simulink library "WECSim_Lib_Body_Elements_2022b"  (R2022b)
settings: Solver=VariableStepAuto  StartTime=0.0  StopTime=10.0  RelTol=1e-3
undefined symbols (not defined in the file or in its folder): body, simu, waves, X, Y, Z
libraries: nesl_utility x24, sm_lib x21, $bdroot x12, vrlib x2
(part 1 of 4)
settings Model: Creator=kmruehl  LastModifiedBy=shusain
settings SolverCC: AlgebraicLoopSolver=TrustRegion
settings DebuggingCC: UnconnectedInputMsg=warning  UnconnectedOutputMsg=warning  UnconnectedLineMsg=warning  SFMachineParentedDataDiag=warning
settings ModelReferenceCC: EnableRefExpFcnMdlSchedulingChecks=on

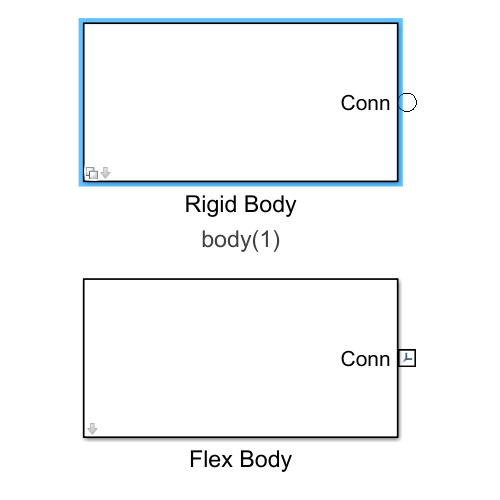
[thumbnail: Simulink's stored preview of the top-level diagram]
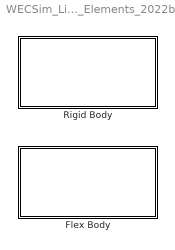
== system WECSim_Lib_Body_Elements_2022b ==
  Flex Body : Subsystem  VariantControl=(default)  mask(Flex Body){body=body(1), InputFileText=Global Reference Frame option "Use Input File" is selected., h5File=hydroData/*.h5, geometryFile=geometry/*.stl, mass=0, inertia=0 0 0, nonHydro=0, nonlinearHydro=0, centerGravity=0 0 0, centerBuoyancy=0 0 0, dof=, volume=0, flex=1, displacement=0 0 0, axis=0 1 0, angle=0, option=0, cd=0 0 0, ca=0 0 0, area=0 0 0, VME=0, rgME=0 0 0, z=0 0 1}
      mask prompts: body "Body Number:"; mass "Body Mass [kg]:"; inertia "MoI [kg*m^2]:"; nonHydro "Nonhydro Body"; nonlinearHydro "Nonlinear Hydrodynamics"; centerGravity "Center of gravity [m]"; centerBuoyancy "Center of buoyancy [m]"; dof "Degrees of freedom"; volume "Displaced Volume [m^3]"; flex "Flexible Body"; displacement "Initial Linear Displacement"; axis "Initial Angular Displacement Axis"; angle "Initial Angular Displacement"; option "On/Off"; cd "Drag coefficient"; ca "Added mass coefficient"; area "Characteristic Area"; VME "Characteristic Volume"; rgME "Point of Application"; z "Z axis"
      mask help:
      | A Flex Body may contain generalized body modes that account for various bending, shear or other deformation modes. The BEM output must contain data for these additional DOFs.
      |
      | The variable name input below must be 'body(i)' where i=1,2,...
      | body(i) must be defined in the input file with the following fields:
      |
      |     .flexHydroBody = 1 (required)
      |             Float.
      |             Flag that creates a flex body. Set equal to 1 if the BEM data contains more than 6 degrees of freedom.
      |     .filename (required)
      |             String.
      |             The file path specifying the .h5 file for the body.
      |     .mass (required)
      |             Float or string.
      |             The translational interia or mass of the body in kg. If a string, the value must be 'equilibrium'. Default = [ ]
      |     .momOfIntertia (required)
      |             3x1 vector [Ixx Iyy Izz].
      |             Rotational intertia of the body in kg*m^2. Default = [ ]
      |     .geometryFile (optional)
      |             String
      |             Path to the geometry file of the body (.stl). Required for nonlinear hydrodynamics or visualization. Default = [ ]
      mask init:
      | if exist('body','var')
      |     % geometry file name
      |     h=[gcb '/Structure/Body Properties'];
      |     geomFile=body.geometryFile;
      |     set_param(h,'ExtGeomFileName',geomFile);
      |     geomType='STL';
      |     % split version e.g. '9.10.0.16028 (R2021a)' into 9, 10, 0, NaN.
      |     % cannot compare str2double('9.10') because it becomes '9.1' 
      |     ver=split(version,'.');
      |     ver=str2double(ver(1:3));
      |     if ver(1) < 9 || (ver(1) == 9 && ver(2) < 6)
      |        set_param(h,'ExtGeomFileType',geomType);
      |     end
      |     % toWorkSpace: outputs
      |     h=[gcb '/To Workspace'];
      |     responseName=['body' num2str(body.number) '_out'];
      |     set_param(h,'VariableName',responseName);
      |     % toWorkSpace: hydrostatic pressures
      |     h=[gcb '/Hydrostatic Restoring Force Calculation/Hydrostatic Restoring Force Calculation/Linear and Nonlinear Restoring Force Variant Subsystem/Nonlinear Hydrostatic Restoring Force/To Workspace1'];
      |     responseName=['body' num2str(body.number) '_hspressure_out'];
      |     set_param(h,'VariableName',responseName); 
      |     % toWorkSpace: wave pressures (nonlinear Froude-Krylov)
      |     h=[gcb '/Wave Diffraction and Excitation Force Calculation/Wave Diffraction and Excitation Force Calculation/Nonlinear FK Force Variant Subsystem/With Nonlinear FroudeKrylov Force/To Workspace'];
      |     responseName=['body' num2str(body.number) '_wavenonlinearpressure_out'];
      |     set_param(h,'VariableName',responseName);
      |     % toWorkSpace: wave pressures (linear Froude-Krylov)
      |     h=[gcb '/Wave Diffraction and Excitation Force Calculation/Wave Diffraction and Excitation Force Calculation/Nonlinear FK Force Variant Subsystem/With Nonlinear FroudeKrylov Force/To Workspace1'];
      |     responseName=['body' num2str(body.number) '_wavelinearpressure_out'];
      |     set_param(h,'VariableName',responseName);
      |     % position: GoTo 
      |     h=[gcb '/Goto'];
      |     responseName=['disp' num2str(body.number)];
      |     set_param(h,'GotoTag',responseName);
      |     % position: From
      |     h=[gcb '/From'];
      |     responseName=['disp' num2str(body.number)];
      |     set_param(h,'GotoTag',responseName);
      |     % velocity: GoTo 
      |     h=[gcb '/Goto1'];
      |     responseName=['vel' num2str(body.number)];
      |     set_param(h,'GotoTag',responseName);
      |     % velocity: From 
      |     h=[gcb '/From1'];
      |     responseName=['vel' num2str(body.number)];
      |     set_param(h,'GotoTag',responseName);
      |     % acceleration: GoTo 
      |     h=[gcb '/Goto2'];
      |     responseName=['acc' num2str(body.number)];
      |     set_param(h,'GotoTag',responseName);
      |     % acceleration: From 
      |     h=[gcb '/From2'];
      |     responseName=['acc' num2str(body.number)];
      |     set_param(h,'GotoTag',responseName);
      |     %%
      |     % Flex Body Morison Element: Off
      |     h = [gcb '/Morrison Element and Viscous Damping Force Calculation/Morison Element and Viscous Damping Force Calculation/Morison Element Variant Subsystem/Morison Element Off'];
      |     responseName = ['sv_b' num2str(body.number) '_MEOff'];
      |     set_param(h,'VariantControl',responseName);
      |     %%
      |     % Flex Body Morison Element: On
      |     h = [gcb '/Morrison Element and Viscous Damping Force Calculation/Morison Element and Viscous Damping Force Calculation/Morison Element Variant Subsystem/Morison Element On'];
      |     responseName = ['sv_b' num2str(body.number) '_MEOn'];
      |     set_param(h,'VariantControl',responseName);
      |     %%
      |     % Flex Body Nonlinear FroudeKrylov Force: Off
      |     h = [gcb '/Wave Diffraction and Excitation Force Calculation/Wave Diffraction and Excitation Force Calculation/Nonlinear FK Force Variant Subsystem/No Nonlinear FroudeKrylov Force'];
      |     responseName = ['sv_b' num2str(body.number) '_linearHydro'];
      |     set_param(h,'VariantControl',responseName);
      |     %%
      |     % Flex Body Nonlinear FroudeKrylov Force: On
      |     h = [gcb '/Wave Diffraction and Excitation Force Calculation/Wave Diffraction and Excitation Force Calculation/Nonlinear FK Force Variant Subsystem/With Nonlinear FroudeKrylov Force'];
      |     responseName = ['sv_b' num2str(body.number) '_nonlinearHydro'];
      |     set_param(h,'VariantControl',responseName);
      |     %%
      |     % Flex Body Nonlinear Restoring: Off
      |     h = [gcb '/Hydrostatic Restoring Force Calculation/Hydrostatic Restoring Force Calculation/Linear and Nonlinear Restoring Force Variant Subsystem/Linear Hydrostatic Restoring Force'];
      |     responseName = ['sv_b' num2str(body.number) '_linearHydro'];
      |     set_param(h,'VariantControl',responseName);
      |     %%
      |     % Flex Body Nonlinear Restoring: On
      |     h = [gcb '/Hydrostatic Restoring Force Calculation/Hydrostatic Restoring Force Calculation/Linear and Nonlinear Restoring Force Variant Subsystem/Nonlinear Hydrostatic Restoring Force'];
      |     responseName = ['sv_b' num2str(body.number) '_nonlinearHydro'];
      |     set_param(h,'VariantControl',responseName);
      |     %%
      |     % Flex Body Nonlinear FroudeKrylov or Restoring: Instantaneous Free Surface
      |     h = [gcb '/Nonlinear Wave Elevation/Linear or Instantaneous Free Surface/Instantaneous Water Free Surface'];
      |     responseName = ['sv_b' num2str(body.number) '_instFS'];
      |     set_param(h,'VariantControl',responseName);
      |     %%
      |     % Flex Body Nonlinear FroudeKrylov or Restoring: Mean Free Surface
      |     h = [gcb '/Nonlinear Wave Elevation/Linear or Instantaneous Free Surface/Mean Water Free Surface'];
      |     responseName = ['sv_b' num2str(body.number) '_meanFS'];
      |     set_param(h,'VariantControl',responseName);
      |     %%
      | end
      mask Help:
      | A Flex Body may contain generalized body modes that account for various bending, shear or other deformation modes. The BEM output must contain data for these additional DOFs.
      | 
      | The variable name input below must be 'body(i)' where i=1,2,...
      | body(i) must be defined in the input file with the following fields:
      | 
      |     .flexHydroBody = 1 (required)
      |             Float.
      |             Flag that creates a flex body. Set equal to 1 if the BEM data contains more than 6 degrees of freedom.
      |     .filename (required)
      |             String.
      |             The file path specifying the .h5 file for the body.
      |     .mass (required)
      |             Float or string.
      |             The translational interia or mass of the body in kg. If a string, the value must be 'equilibrium'. Default = [ ]
      |     .momOfIntertia (required)
      |             3x1 vector [Ixx Iyy Izz].
      |             Rotational intertia of the body in kg*m^2. Default = [ ]
      |     .geometryFile (optional)
      |             String
      |             Path to the geometry file of the body (.stl). Required for nonlinear hydrodynamics or visualization. Default = [ ]
      mask TypeOptions nonHydro: 0 | 1 | 2
      mask Callback nonHydro: bodyClassCallback(gcbh)
      mask TypeOptions nonlinearHydro: 0 | 1 | 2
      mask TypeOptions flex: 0 | 1
      mask TypeOptions option: 0 | 1 | 2
      mask Callback option: bodyClassCallback(gcbh)
      mask DialogControl CustomParameterGroup Prompt: Custom Parameters
      mask DialogControl std_opts Prompt: Standard Options
      mask DialogControl H5button Prompt: Select .h5 File
      mask DialogControl H5button Callback: h5ButtonCallback(gcbh)
      mask DialogControl STLbutton Prompt: Select .stl File
      mask DialogControl STLbutton Callback: stlButtonCallback(gcbh)
      mask DialogControl inertia Tooltip: Moment of Inertia
      mask DialogControl initial Prompt: Initial Displacement
      mask DialogControl morisonElement Prompt: Morison Element
      mask DialogControl rgME Tooltip: The vector from the body COG to point of application for the Morison Element
      mask DialogControl z Tooltip: The unit normal vector center axis of the Morison Element
  Rigid Body : Subsystem  Variant=on  AllowZeroVariantControls=on  mask(Rigid Body){body=body(1), InputFileText=Global Reference Frame option "Use Input File" is selected., h5File=hydroData/*.h5, geometryFile=geometry/*.stl, mass=0, inertia=0 0 0, nonHydro=0, nonlinearHydro=0, centerGravity=0 0 0, centerBuoyancy=0 0 0, dof=6, volume=0, flex=0, displacement=0 0 0, axis=0 1 0, angle=0, option=0, cd=0 0 0, ca=0 0 0, area=0 0 0, VME=0, rgME=0 0 0, z=0 0 1}
      mask prompts: body "Body Number:"; mass "Body Mass [kg]:"; inertia "MoI [kg*m^2]:"; nonHydro "Nonhydro Body"; nonlinearHydro "Nonlinear Hydrodynamics"; centerGravity "Center of gravity [m]"; centerBuoyancy "Center of buoyancy [m]"; dof "Degrees of freedom"; volume "Displaced Volume [m^3]"; flex "Flexible Body"; displacement "Initial Linear Displacement"; axis "Initial Angular Displacement Axis"; angle "Initial Angular Displacement"; option "On/Off"; cd "Drag coefficient"; ca "Added mass coefficient"; area "Characteristic Area"; VME "Characteristic Volume"; rgME "Point of Application"; z "Z axis"
      mask help:
      | A rigid body has no generalized body modes. It can be a standard hydrodynamic body, a drag body, or a non-hydrodynamic body.
      |
      | The variable name input below must be 'body(i)' where i=1,2,...
      | body(i) must be defined in the input file with the fields appropriate to each variant.
      mask init:
      | if exist('body','var')
      |     %%
      |     % Hydro Body
      |     h = [gcb '/Hydrodynamic Body'];
      |     responseName = ['sv_b' num2str(body.number) '_hydroBody'];
      |     set_param(h,'VariantControl',responseName);
      |     %%
      |     % Hydro Body Morison Element: Off
      |     h = [gcb '/Hydrodynamic Body/Morison Element and Viscous Damping Force Calculation/Morison Element Variant Subsystem/Morison Element Off'];
      |     responseName = ['sv_b' num2str(body.number) '_MEOff'];
      |     set_param(h,'VariantControl',responseName);
      |     %%
      |     % Hydro Body Morison Element: On
      |     h = [gcb '/Hydrodynamic Body/Morison Element and Viscous Damping Force Calculation/Morison Element Variant Subsystem/Morison Element On'];
      |     responseName = ['sv_b' num2str(body.number) '_MEOn'];
      |     set_param(h,'VariantControl',responseName);
      |     %%
      |     % Hydro Body Nonlinear Froude Krylov Force: Off
      |     h = [gcb '/Hydrodynamic Body/Wave Diffraction and Excitation Force Calculation/Nonlinear FK Force Variant Subsystem/No Nonlinear FroudeKrylov Force'];
      |     responseName = ['sv_b' num2str(body.number) '_linearHydro'];
      |     set_param(h,'VariantControl',responseName);
      |     %%
      |     % Hydro Body Nonlinear Froude Krylov Force: On
      |     h = [gcb '/Hydrodynamic Body/Wave Diffraction and Excitation Force Calculation/Nonlinear FK Force Variant Subsystem/With Nonlinear FroudeKrylov Force'];
      |     responseName = ['sv_b' num2str(body.number) '_nonlinearHydro'];
      |     set_param(h,'VariantControl',responseName);
      |     %%
      |     % Hydro Body Nonlinear Restoring: Off
      |     h = [gcb '/Hydrodynamic Body/Hydrostatic Restoring Force Calculation/Linear and Nonlinear Restoring Force Variant Subsystem/Linear Hydrostatic Restoring Force'];
      |     responseName = ['sv_b' num2str(body.number) '_linearHydro'];
      |     set_param(h,'VariantControl',responseName);
      |     %%
      |     % Hydro Body Nonlinear Restoring: On
      |     h = [gcb '/Hydrodynamic Body/Hydrostatic Restoring Force Calculation/Linear and Nonlinear Restoring Force Variant Subsystem/Nonlinear Hydrostatic Restoring Force'];
      |     responseName = ['sv_b' num2str(body.number) '_nonlinearHydro'];
      |     set_param(h,'VariantControl',responseName);
      |     %%
      |     
      |     % Hydro Body Regular Excitation Passive Yaw: Off
      |     h = [gcb '/Hydrodynamic Body/Wave Diffraction and Excitation Force Calculation/Linear Wave Excitation Force Variant Subsystem'];
      |     responseName = ['regularWaves_b' num2str(body.number)];
      |     set_param(h,'VariantControl',responseName);
      |     %%
      |     % Hydro Body Regular Excitation Passive Yaw: On
      |     h = [gcb '/Hydrodynamic Body/Wave Diffraction and Excitation Force Calculation/Linear Wave Excitation Force Variant Subsystem'];
      |     responseName = ['sv_regularWavesNonLinYaw_b' num2str(body.number)];
      |     set_param(h,'VariantControl',responseName);
      |     %%    
      |     % Hydro Body Irregular Excitation Passive Yaw: Off
      |     h = [gcb '/Hydrodynamic Body/Wave Diffraction and Excitation Force Calculation/Linear Wave Excitation Force Variant Subsystem'];
      |     responseName = ['sv_irregularWaves_b' num2str(body.number)];
      |     set_param(h,'VariantControl',responseName);
      |     %%
      |     % Hydro Body Irregular Excitation Passive Yaw: On
      |     h = [gcb '/Hydrodynamic Body/Wave Diffraction and Excitation Force Calculation/Linear Wave Excitation Force Variant Subsystem'];
      |     responseName = ['sv_irregularWavesNonLinYaw_b' num2str(body.number)];
      |     set_param(h,'VariantControl',responseName);
      |     %%        
      |     
      |     % Hydro Body Nonlinear Froude Krylov or Restoring: Instantaneous Free Surface
      |     h = [gcb '/Hydrodynamic Body/Nonlinear Wave Elevation/Linear or Instantaneous Free Surface/Instantaneous Water Free Surface'];
      |     responseName = ['sv_b' num2str(body.number) '_instFS'];
      |     set_param(h,'VariantControl',responseName);
      |     %%
      |     % Hydro Body Nonlinear Froude Krylov or Restoring: Mean Free Surface
      |     h = [gcb '/Hydrodynamic Body/Nonlinear Wave Elevation/Linear or Instantaneous Free Surface/Mean Water Free Surface'];
      |     responseName = ['sv_b' num2str(body.number) '_meanFS'];
      |     set_param(h,'VariantControl',responseName);
      |     %%
      |     % Non-Hydro Body
      |     h = [gcb '/Non-Hydro Body'];
      |     responseName = ['sv_b' num2str(body.number) '_nonHydroBody'];
      |     set_param(h,'VariantControl',responseName);
      |     %%
      |     % Drag Body
      |     h = [gcb '/Drag Body'];
      |     responseName = ['sv_b' num2str(body.number) '_dragBody'];
      |     set_param(h,'VariantControl',responseName);
      |     %%
      |     % Drag Body Morison Element: Off
      |     h = [gcb '/Drag Body/Morison Element and Viscous Damping Force Calculation/Morison Element Variant Subsystem/Morison Element Off'];
      |     responseName = ['sv_b' num2str(body.number) '_MEOff'];
      |     set_param(h,'VariantControl',responseName);
      |     %%
      |     % Drag Body Morison Element: On
      |     h = [gcb '/Drag Body/Morison Element and Viscous Damping Force Calculation/Morison Element Variant Subsystem/Morison Element On'];
      |     responseName = ['sv_b' num2str(body.number) '_MEOn'];
      |     set_param(h,'VariantControl',responseName);
      |     %%
      |     % Set zero active variant controls to prevent label issue
      |     set_param(gcb,'AllowZeroVariantControls','on');
      | end
      | clear bc h geomFile responseName
      settings: AttributesFormatString=%<body>
      mask Help:
      | A rigid body has no generalized body modes. It can be a standard hydrodynamic body, a drag body, or a non-hydrodynamic body.
      | 
      | The variable name input below must be 'body(i)' where i=1,2,...
      | body(i) must be defined in the input file with the fields appropriate to each variant.
      mask TypeOptions nonHydro: 0 | 1 | 2
      mask Callback nonHydro: bodyClassCallback(gcbh)
      mask TypeOptions nonlinearHydro: 0 | 1 | 2
      mask TypeOptions flex: 0 | 1
      mask TypeOptions option: 0 | 1 | 2
      mask Callback option: bodyClassCallback(gcbh)
      mask DialogControl CustomParameterGroup Prompt: Custom Parameters
      mask DialogControl std_opts Prompt: Standard Options
      mask DialogControl H5button Prompt: Select .h5 File
      mask DialogControl H5button Callback: h5ButtonCallback(gcbh)
      mask DialogControl STLbutton Prompt: Select .stl File
      mask DialogControl STLbutton Callback: stlButtonCallback(gcbh)
      mask DialogControl inertia Tooltip: Moment of Inertia
      mask DialogControl initial Prompt: Initial Displacement
      mask DialogControl morisonElement Prompt: Morison Element
      mask DialogControl rgME Tooltip: The vector from the body COG to point of application for the Morison Element
      mask DialogControl z Tooltip: The unit normal vector center axis of the Morison Element

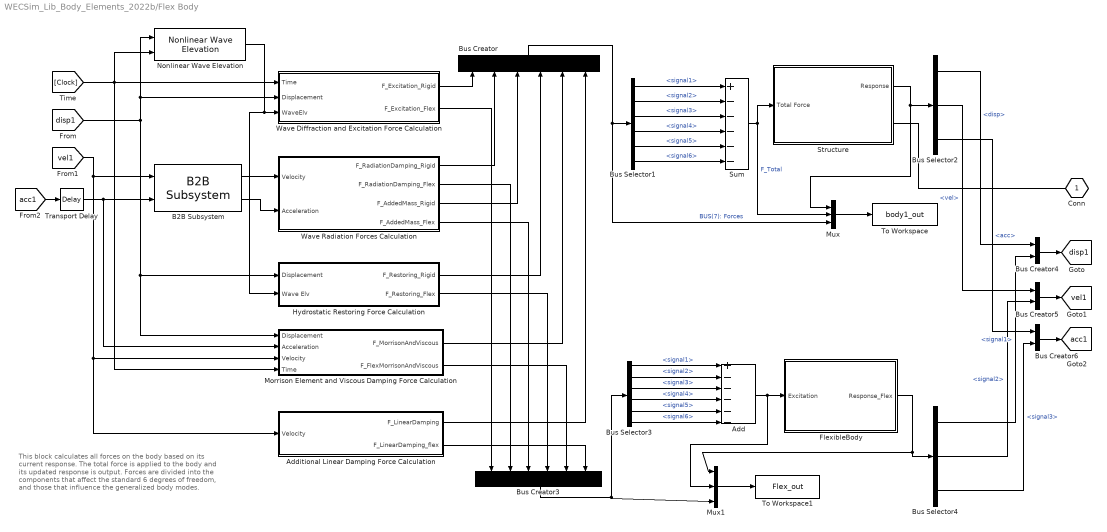
== system WECSim_Lib_Body_Elements_2022b/Flex Body ==
  note: This block calculates all forces on the body based on its current response. The total force is applied to the body and its updated response is output.
      |
      | Forces are divided into the components that affect the standard 6 degrees of freedom, and those that influence the generalized body modes.
  Add : Sum  Inputs=+-----
  Additional Linear Damping Force Calculation : Subsystem
  B2B Subsystem : $bdroot/Rigid Body/Hydrodynamic Body/B2B Subsystem  SystemSampleTime=-1  Latency=0  AutoFrameSizeCalculation=off
  Bus Creator : BusCreator  Inputs=6
  Bus Creator3 : BusCreator  Inputs=6
  Bus Creator4 : BusCreator  Inputs=2
  Bus Creator5 : BusCreator  Inputs=2
  Bus Creator6 : BusCreator  Inputs=2
  Bus Selector1 : BusSelector  OutputSignals=signal1,signal2,signal3,signal4,signal5,signal6
  Bus Selector2 : BusSelector  OutputSignals=disp,vel,acc
  Bus Selector3 : BusSelector  OutputSignals=signal1,signal2,signal3,signal4,signal5,signal6
  Bus Selector4 : BusSelector  OutputSignals=signal1,signal2,signal3
  FlexibleBody : Subsystem
  Hydrostatic Restoring Force Calculation : Subsystem
  Morrison Element and Viscous Damping Force Calculation : Subsystem
  Mux : Mux  Inputs=3
  Mux1 : Mux  Inputs=3
  Nonlinear Wave Elevation : $bdroot/Rigid Body/Hydrodynamic Body/Nonlinear Wave Elevation  SystemSampleTime=simu.nonlinearDt  Latency=0  AutoFrameSizeCalculation=off
  Structure : Subsystem
  Sum : Sum  Inputs=+-----
  To Workspace : ToWorkspace  VariableName=body1_out  SaveFormat=Structure With Time  SampleTime=simu.dtOut
  To Workspace1 : ToWorkspace  VariableName=Flex_out  SaveFormat=Structure With Time  SampleTime=simu.dtOut
  Transport Delay : TransportDelay  DelayTime=10e-8
  Wave Diffraction and Excitation Force Calculation : Subsystem
  Wave Radiation Forces Calculation : Subsystem
  Conn : PMIOPort  Side=Right
  tag scope: acc1=global, disp1=global, vel1=global
  wires:
  Bus Creator/1 -> Mux/3, Bus Selector1/1  "BUS(7): Forces"
  Structure/1(Response) -> Mux/1, Bus Selector2/1
  Sum/1 -> Mux/2, Structure/1(Total Force)  "F_Total"
  Mux/1 -> To Workspace/1
  Bus Selector1/4 -> Sum/4  "<signal4>"
  Bus Selector1/3 -> Sum/3  "<signal3>"
  Bus Selector1/5 -> Sum/5  "<signal5>"
  Bus Selector1/2 -> Sum/2  "<signal2>"
  Bus Selector1/1 -> Sum/1  "<signal1>"
  Bus Selector1/6 -> Sum/6  "<signal6>"
  [vel1] -> Additional Linear Damping Force Calculation/1(Velocity), Morrison Element and Viscous Damping Force Calculation/3(Velocity), B2B Subsystem/1
  B2B Subsystem/2 -> Wave Radiation Forces Calculation/2(Acceleration)
  B2B Subsystem/1 -> Wave Radiation Forces Calculation/1(Velocity)
  [disp1] -> Nonlinear Wave Elevation/1, Wave Diffraction and Excitation Force Calculation/2(Displacement), Morrison Element and Viscous Damping Force Calculation/1(Displacement), Hydrostatic Restoring Force Calculation/1(Displacement)
  Nonlinear Wave Elevation/1 -> Hydrostatic Restoring Force Calculation/2(Wave Elv), Wave Diffraction and Excitation Force Calculation/3(WaveElv)
  Hydrostatic Restoring Force Calculation/1(F_Restoring_Rigid) -> Bus Creator/4
  Wave Radiation Forces Calculation/1(F_RadiationDamping_Rigid) -> Bus Creator/2
  Wave Diffraction and Excitation Force Calculation/1(F_Excitation_Rigid) -> Bus Creator/1
  Wave Radiation Forces Calculation/3(F_AddedMass_Rigid) -> Bus Creator/3
  [Clock] -> Nonlinear Wave Elevation/2, Morrison Element and Viscous Damping Force Calculation/4(Time), Wave Diffraction and Excitation Force Calculation/1(Time)
  Mux1/1 -> To Workspace1/1
  Wave Diffraction and Excitation Force Calculation/2(F_Excitation_Flex) -> Bus Creator3/1
  Wave Radiation Forces Calculation/2(F_RadiationDamping_Flex) -> Bus Creator3/2
  Wave Radiation Forces Calculation/4(F_AddedMass_Flex) -> Bus Creator3/3
  Bus Creator3/1 -> Bus Selector3/1, Mux1/3
  Bus Selector3/1 -> Add/1  "<signal1>"
  Bus Selector3/2 -> Add/2  "<signal2>"
  Bus Selector3/3 -> Add/3  "<signal3>"
  Bus Selector3/4 -> Add/4  "<signal4>"
  Add/1 -> Mux1/2, FlexibleBody/1(Excitation)
  FlexibleBody/1(Response_Flex) -> Bus Selector4/1, Mux1/1
  Bus Selector4/1 -> Bus Creator4/2  "<signal1>"
  Bus Selector4/2 -> Bus Creator5/2  "<signal2>"
  Bus Selector4/3 -> Bus Creator6/2  "<signal3>"
  Additional Linear Damping Force Calculation/1(F_LinearDamping) -> Bus Creator/6
  Morrison Element and Viscous Damping Force Calculation/2("F_FlexMorrisonAndViscous ") -> Bus Creator3/5
  Bus Selector3/5 -> Add/5  "<signal5>"
  Additional Linear Damping Force Calculation/2(F_LinearDamping_flex) -> Bus Creator3/6
  Bus Selector3/6 -> Add/6  "<signal6>"
  Bus Selector2/1 -> Bus Creator4/1  "<disp>"
  Bus Creator4/1 -> [disp1]
  Bus Creator5/1 -> [vel1]
  Bus Creator6/1 -> [acc1]
  Bus Selector2/2 -> Bus Creator5/1  "<vel>"
  Bus Selector2/3 -> Bus Creator6/1  "<acc>"
  Hydrostatic Restoring Force Calculation/2(F_Restoring_Flex) -> Bus Creator3/4
  Morrison Element and Viscous Damping Force Calculation/1(F_MorrisonAndViscous) -> Bus Creator/5
  [acc1] -> Transport Delay/1
  Transport Delay/1 -> B2B Subsystem/2, Morrison Element and Viscous Damping Force Calculation/2(Acceleration)
  connections:
  Conn/RConn1 -- Structure/RConn1

== system WECSim_Lib_Body_Elements_2022b/Rigid Body ==
  note: 1) Add Subsystem or Model blocks as valid variant choices.
      | 2) You cannot connect blocks at this level. At simulation, connectivity is automatically
      | determined, based on the active variant and port name matching.
  Drag Body : Subsystem  VariantControl=sv_b1_dragBody  mask(Drag Body){body=body}
      mask prompts: body "Body Name:"
      mask help:
      | A drag body contains six degrees of freedom in x, y, z and Mx, My, Mz. It contains a buoyant force, linear damping force, and Morison Element and viscous forces. It is not influenced by wave excitation, radiation damping or radiation added mass.
      |
      | The variable name input below must be 'body(i)' where i=1,2,...
      | body(i) must be defined in the input file with the following fields:
      |
      |     .mass (required)
      |             Float or string.
      |             The translational interia or mass of the body in kg. If a string, the value must be 'equilibrium'. Default = [ ]
      |     .momOfIntertia (required)
      |             3x1 vector [Ixx Iyy Izz].
      |             Rotational intertia of the body in kg*m^2. Default = [ ]
      |     .filename (required)
      |             String.
      |             The file path specifying the .h5 file for the body.
      |     .name (optional)
      |             String.
      |             Specifies the body name. Default = [ ]
      |     .cg (optional)
      |             3x1 float vector [x y z]
      |     .cb (optional)
      |             3x1 float vector [x y z]
      |             Body center of buoyancy in m. Default = [ ].
      |     .dispVol (optional)
      |             Float.
      |             Displaced volume at the equilibrium position in m^3. Default = [ ]
      |     .geometryFile (optional)
      |             String
      |             Path to the geometry file of the body (.stl). Required for nonlinear hydrodynamics or visualization. Default = [ ]
      mask init:
      | if exist('body','var')
      |     % geometry file name
      |     h=[gcb '/Structure/Body Properties'];
      |     geomFile=body.geometryFile;
      |     set_param(h,'ExtGeomFileName',geomFile);
      |     geomType='STL';
      |     % split version e.g. '9.10.0.16028 (R2021a)' into 9, 10, 0, NaN.
      |     % cannot compare str2double('9.10') because it becomes '9.1' 
      |     ver=split(version,'.');
      |     ver=str2double(ver(1:3));
      |     if ver(1) < 9 || (ver(1) == 9 && ver(2) < 6)
      |        set_param(h,'ExtGeomFileType',geomType);
      |     end
      |     % toWorkSpace: outputs
      |     h=[gcb '/To Workspace'];
      |     responseName=['body' num2str(body.number) '_out'];
      |     set_param(h,'VariableName',responseName);
      |     % position GoTo 
      |     h=[gcb '/Goto'];
      |     responseName=['disp' num2str(body.number)];
      |     set_param(h,'GotoTag',responseName);
      |     % position From
      |     h=[gcb '/From'];
      |     responseName=['disp' num2str(body.number)];
      |     set_param(h,'GotoTag',responseName);
      |     % velocity GoTo 
      |     h=[gcb '/Goto1'];
      |     responseName=['vel' num2str(body.number)];
      |     set_param(h,'GotoTag',responseName);
      |     % velocity From 
      |     h=[gcb '/From1'];
      |     responseName=['vel' num2str(body.number)];
      |     set_param(h,'GotoTag',responseName);
      |     % acceleration GoTo 
      |     h=[gcb '/Goto2'];
      |     responseName=['acc' num2str(body.number)];
      |     set_param(h,'GotoTag',responseName);
      |     % acceleration From 
      |     h=[gcb '/From2'];
      |     responseName=['acc' num2str(body.number)];
      |     set_param(h,'GotoTag',responseName);
      | end
  Hydrodynamic Body : Subsystem  VariantControl=sv_b1_hydroBody  mask(Hydrodynamic Body){body=body, waveGroup=waves.waveGroup}
      mask prompts: body "Body Name:"; waveGroup "Wave Group:"
      mask help:
      | A Hydrodynamic Body contains six degrees of freedom in x, y, z and Mx, My, Mz. All wave forces interact with a hydrodynamic body.
      |
      | The variable name input below must be 'body(i)' where i=1,2,...
      | body(i) must be defined in the input file with the following fields:
      |
      |     .filename (required)
      |             String.
      |             The file path specifying the .h5 file for the body.
      |     .mass (required)
      |             Float or string.
      |             The translational interia or mass of the body in kg. If a string, the value must be 'equilibrium'. Default = [ ]
      |     .momOfIntertia (required)
      |             3x1 vector [Ixx Iyy Izz].
      |             Rotational intertia of the body in kg*m^2. Default = [ ]
      |     .geometryFile (optional)
      |             String
      |             Path to the geometry file of the body (.stl). Required for nonlinear hydrodynamics or visualization. Default = [ ]
      mask init:
      | if exist('body','var')
      |     % geometry file name
      |     h=[gcb '/Structure/Body Properties'];
      |     geomFile=body.geometryFile;
      |     set_param(h,'ExtGeomFileName',geomFile);
      |     geomType='STL';
      |     % split version e.g. '9.10.0.16028 (R2021a)' into 9, 10, 0, NaN.
      |     % cannot compare str2double('9.10') because it becomes '9.1' 
      |     ver=split(version,'.');
      |     ver=str2double(ver(1:3));
      |     if ver(1) < 9 || (ver(1) == 9 && ver(2) < 6)
      |        set_param(h,'ExtGeomFileType',geomType);
      |     end
      |     % toWorkSpace: outputs
      |     h=[gcb '/To Workspace'];
      |     responseName=['body' num2str(body.number) '_out'];
      |     set_param(h,'VariableName',responseName);
      |     % toWorkSpace: hydrostatic pressures
      |     h=[gcb '/Hydrostatic Restoring Force Calculation/Linear and Nonlinear Restoring Force Variant Subsystem/Nonlinear Hydrostatic Restoring Force/To Workspace1'];
      |     responseName=['body' num2str(body.number) '_hspressure_out'];
      |     set_param(h,'VariableName',responseName); 
      |     % toWorkSpace: wave pressures (non-linear Freude-Krylov)
      |     h=[gcb '/Wave Diffraction and Excitation Force Calculation/Nonlinear FK Force Variant Subsystem/With Nonlinear FroudeKrylov Force/To Workspace'];
      |     responseName=['body' num2str(body.number) '_wavenonlinearpressure_out'];
      |     set_param(h,'VariableName',responseName);
      |     % toWorkSpace: wave pressures (linear Freude-Krylov)
      |     h=[gcb '/Wave Diffraction and Excitation Force Calculation/Nonlinear FK Force Variant Subsystem/With Nonlinear FroudeKrylov Force/To Workspace1'];
      |     responseName=['body' num2str(body.number) '_wavelinearpressure_out'];
      |     set_param(h,'VariableName',responseName);
      |     % position GoTo 
      |     h=[gcb '/Goto'];
      |     responseName=['disp' num2str(body.number)];
      |     set_param(h,'GotoTag',responseName);
      |     % position From
      |     h=[gcb '/From'];
      |     responseName=['disp' num2str(body.number)];
      |     set_param(h,'GotoTag',responseName);
      |     % velocity GoTo 
      |     h=[gcb '/Goto1'];
      |     responseName=['vel' num2str(body.number)];
      |     set_param(h,'GotoTag',responseName);
      |     % velocity From 
      |     h=[gcb '/From1'];
      |     responseName=['vel' num2str(body.number)];
      |     set_param(h,'GotoTag',responseName);
      |     % acceleration GoTo 
      |     h=[gcb '/Goto2'];
      |     responseName=['acc' num2str(body.number)];
      |     set_param(h,'GotoTag',responseName);
      |     % acceleration From 
      |     h=[gcb '/From2'];
      |     responseName=['acc' num2str(body.number)];
      |     set_param(h,'GotoTag',responseName);
      | end
  Non-Hydro Body : Subsystem  VariantControl=sv_b1_nonHydroBody  mask(Non-hydrodynamic body){body=body}
      mask prompts: body "Body Name:"
      mask help:
      | A non-hydrodynamic Body contains six degrees of freedom in x, y, z and Mx, My, Mz. It is not influenced by wave forces and does not radiate a wave. Only the buoyant force acts on a non-hydrodynamic body.
      |
      | The variable name input below must be 'body(i)' where i=1,2,...
      | body(i) must be defined in the input file with the following fields:
      |
      |     .nhBody = 1 (required)
      |             Float.
      |             Flag that marks the body as non-hydrodynamic. Must be 1 for a non-hydrodynamic body. Default = 0
      |     .mass (required)
      |             Float or string.
      |             The translational interia or mass of the body in kg. If a string, the value must be 'equilibrium'. Default = [ ]
      |     .momOfIntertia (required)
      |             3x1 vector [Ixx Iyy Izz].
      |             Rotational intertia of the body in kg*m^2. Default = [ ]
      |     .filename (optional)
      |             String.
      |             The file path specifying the .h5 file for the body.
      |     .name (optional)
      |             String.
      |             Specifies the body name. Default = [ ]
      |     .cg (optional)
      |             3x1 float vector [x y z]
      |     .cb (optional)
      |             3x1 float vector [x y z]
      |             Body center of buoyancy in m. Default = [ ].
      |     .dispVol (optional)
      |             Float.
      |             Displaced volume at the equilibrium position in m^3. Default = [ ]
      |     .geometryFile (optional)
      |             String
      |             Path to the geometry file of the body (.stl). Required for nonlinear hydrodynamics or visualization. Default = [ ]
      mask init:
      | if exist('body','var')
      |     % geometry file name
      |     h=[gcb '/Structure/Body Properties'];
      |     geomFile=body.geometryFile;
      |     set_param(h,'ExtGeomFileName',geomFile);
      |     geomType='STL';
      |     % split version e.g. '9.10.0.16028 (R2021a)' into 9, 10, 0, NaN.
      |     % cannot compare str2double('9.10') because it becomes '9.1' 
      |     ver=split(version,'.');
      |     ver=str2double(ver(1:3));
      |     if ver(1) < 9 || (ver(1) == 9 && ver(2) < 6)
      |        set_param(h,'ExtGeomFileType',geomType);
      |     end
      |     % toWorkSpace: outputs
      |     h=[gcb '/To Workspace'];
      |     responseName=['body' num2str(body.number) '_out'];
      |     set_param(h,'VariableName',responseName);
      | end
  Conn : PMIOPort  Side=Right

== system WECSim_Lib_Body_Elements_2022b/Flex Body/Additional Linear Damping Force Calculation ==
  Velocity : Inport
  Additional Linear Damping Force Calculation : $bdroot/Rigid Body/Hydrodynamic Body/Additional Linear Damping Force Calculation  SystemSampleTime=-1  Latency=0  AutoFrameSizeCalculation=off
  Selector : Selector  InputPortWidth=body.dof  IndexOptions=Index vector (dialog)  Indices=[1:6]  OutputSizes=1
  Selector1 : Selector  InputPortWidth=body.dof  IndexOptions=Index vector (dialog)  Indices=[7:body.dofEnd]  OutputSizes=1
  F_LinearDamping : Outport  PortDimensions=6
  F_LinearDamping_flex : Outport  Port=2  PortDimensions=body.gbmDOF
  wires:
  Selector/1 -> F_LinearDamping/1
  Selector1/1 -> F_LinearDamping_flex/1
  Velocity/1 -> Additional Linear Damping Force Calculation/1  "v"
  Additional Linear Damping Force Calculation/1 -> Selector/1, Selector1/1

== system WECSim_Lib_Body_Elements_2022b/Flex Body/FlexibleBody ==
  note: This block solves the governing equations of motion for the flexible degrees of freedom (generalized body modes) using the flex force components. The response of the generalied body modes is output.
  Excitation : Inport
  Add : Sum  Inputs=--+
  Added Mass Matrix1 : Constant  Value=body.hydroForce.gbm.stiffness
  Added Mass Matrix2 : Constant  Value=body.hydroForce.gbm.damping
  Added Mass Matrix3 : Constant  Value=body.hydroForce.gbm.mass_ff_inv
  Added Mass Matrix4 : Constant  Value=body.hydroForce.gbm.mass_ff_inv
  Bus Creator : BusCreator  Inputs=3
  GBM : StateSpace  A=body.hydroForce.gbm.state_space.A  B=body.hydroForce.gbm.state_space.B  C=body.hydroForce.gbm.state_space.C  D=body.hydroForce.gbm.state_space.D  InitialCondition=0
  Mux : Mux  Inputs=2
  Product1 : Product  Multiplication=Matrix(*)
  Product2 : Product  Multiplication=Matrix(*)
  Product4 : Product  Multiplication=Matrix(*)
  acceleration : Product  Multiplication=Matrix(*)
  displacement : Selector  InputPortWidth=body.gbmDOF*2  IndexOptions=Index vector (dialog)  Indices=[1:body.gbmDOF]  OutputSizes=1
  unit matrix : Constant  Value=zeros(body.gbmDOF,1)
  velocity : Selector  InputPortWidth=2*body.gbmDOF  IndexOptions=Index vector (dialog)  Indices=[body.gbmDOF+1:2*body.gbmDOF]  OutputSizes=1
  Response_Flex : Outport
  wires:
  Excitation/1 -> Product4/2, Add/3
  GBM/1 -> displacement/1, velocity/1
  displacement/1 -> Product1/2, Bus Creator/1
  velocity/1 -> Product2/2, Bus Creator/2
  Added Mass Matrix1/1 -> Product1/1
  Added Mass Matrix2/1 -> Product2/1
  Product1/1 -> Add/1  "F_AddedMass"
  Added Mass Matrix3/1 -> acceleration/1
  Add/1 -> acceleration/2
  Product2/1 -> Add/2
  unit matrix/1 -> Mux/1
  Added Mass Matrix4/1 -> Product4/1
  Product4/1 -> Mux/2
  Mux/1 -> GBM/1
  Bus Creator/1 -> Response_Flex/1
  acceleration/1 -> Bus Creator/3

== system WECSim_Lib_Body_Elements_2022b/Flex Body/Hydrostatic Restoring Force Calculation ==
  note: Do not link the `Hydrostatic Restoring Force Calculation`
      | to the rigid body block, this will break the Flex Body block.
  Displacement : Inport
  Wave Elv : Inport  Port=2
  Hydrostatic Restoring Force Calculation : Subsystem
  Selector : Selector  InputPortWidth=body.dof  IndexOptions=Index vector (dialog)  Indices=[1:6]  OutputSizes=1
  Selector1 : Selector  InputPortWidth=body.dof  IndexOptions=Index vector (dialog)  Indices=[7:body.dofEnd]  OutputSizes=1
  F_Restoring_Rigid : Outport  PortDimensions=6
  F_Restoring_Flex : Outport  Port=2  PortDimensions=body.gbmDOF
  wires:
  Hydrostatic Restoring Force Calculation/1(F_Restoring) -> Selector1/1, Selector/1  "F_Restoring"
  Selector/1 -> F_Restoring_Rigid/1
  Selector1/1 -> F_Restoring_Flex/1
  Displacement/1 -> Hydrostatic Restoring Force Calculation/1(Displacement)  "x"
  Wave Elv/1 -> Hydrostatic Restoring Force Calculation/2(Wave Elv)

== system WECSim_Lib_Body_Elements_2022b/Flex Body/Morrison Element and Viscous Damping Force Calculation ==
  Displacement : Inport
  Acceleration : Inport  Port=2
  Velocity : Inport  Port=3
  Time : Inport  Port=4
  Morison Element and Viscous Damping Force Calculation : $bdroot/Rigid Body/Hydrodynamic Body/Morison Element and Viscous Damping Force Calculation  SystemSampleTime=-1  Latency=0  AutoFrameSizeCalculation=off
  Selector : Selector  InputPortWidth=body.dof  IndexOptions=Index vector (dialog)  Indices=[1:6]  OutputSizes=1
  Selector1 : Selector  InputPortWidth=body.dof  IndexOptions=Index vector (dialog)  Indices=[7:body.dofEnd]  OutputSizes=1
  F_MorrisonAndViscous : Outport  PortDimensions=6
  "F_FlexMorrisonAndViscous " : Outport  Port=2  PortDimensions=body.gbmDOF
  wires:
  Acceleration/1 -> Morison Element and Viscous Damping Force Calculation/2
  Time/1 -> Morison Element and Viscous Damping Force Calculation/4
  Displacement/1 -> Morison Element and Viscous Damping Force Calculation/1
  Velocity/1 -> Morison Element and Viscous Damping Force Calculation/3
  Morison Element and Viscous Damping Force Calculation/1 -> Selector1/1, Selector/1
  Selector/1 -> F_MorrisonAndViscous/1
  Selector1/1 -> "F_FlexMorrisonAndViscous "/1

== system WECSim_Lib_Body_Elements_2022b/Flex Body/Structure ==
  note: Apply the total force to the body and calculate its response relative to the global reference frame.
      |
      | Output force to apply to another body.
  Total Force : Inport
  Body Properties : sm_lib/Body Elements/File Solid  ExtGeomFileName=../geometry/flap.stl  UnitType=Custom  ExtGeomFileUnits=m  StepReaderType=HEX  ExportConvexHullGeometry=off  InertiaType=Custom  Mass=body.mass  MassUnits=kg  CenterOfMass=[0 0 0]  CenterOfMassUnits=m  MomentsOfInertia=body.inertia  MomentsOfInertiaUnits=kg*m^2  ProductsOfInertia=[0 0 0]  ProductsOfInertiaUnits=kg*m^2  BasedOnType=Density  Density=1000  DensityUnits=kg/(m^3)  DoExposeReferenceFrame=on  SerializedFrames=<Frames/>  GraphicType=FromGeometry  MarkerShape=Sphere  MarkerSize=10  MarkerSizeUnits=m  GraphicVisPropType=SimpleVisualProperties  GraphicDiffuseColor=body.viz.color  GraphicSpecularColor=[0.5 0.5 0.5 1.0]  GraphicAmbientColor=[0.15 0.15 0.15 1.0]  GraphicEmissiveColor=[0.0 0.0 0.0 1.0]  GraphicShininess=75  GraphicOpacity=body.viz.opacity
  External Force and Torque : sm_lib/Forces and Torques/External Force and Torque  ForceResolutionFrame=World  EnableForceX=off  EnableForceY=off  EnableForceZ=off  EnableForce=on  TorqueResolutionFrame=World  EnableTorqueX=off  EnableTorqueY=off  EnableTorqueZ=off  EnableTorque=on
  Motion Sensor : $bdroot/Rigid Body/Hydrodynamic Body/Structure/Motion Sensor  SystemSampleTime=-1  VariantActivationTime=update diagram  Latency=0  AutoFrameSizeCalculation=off
  Rigid Transform (Setup CG) : sm_lib/Frames and Transforms/Rigid Transform  TranslationMethod=Cartesian  TranslationStandardOffset=0  TranslationLengthUnit=m  TranslationStandardAxis=+Z  TranslationCartesianOffset=body.centerGravity  TranslationROffset=0  TranslationROffsetUnits=m  TranslationZOffset=0  TranslationZOffsetUnits=m  TranslationThetaOffset=0  TranslationThetaOffsetUnits=deg  RotationMethod=None  RotationAngleUnits=rad  RotationStandardAxis=+Y  RotationAngle=0.05  RotationArbitraryAxis=[0.57735026918962584 0.57735026918962584 0.57735026918962584]  FollAlignAxisA=+X  BaseAlignAxisA=+Y  FollAlignAxisB=+Y  BaseAlignAxisB=+Z  RotationSequenceAxes=FollowerAxes  RotationSequence=XYX  RotationSequenceAngles=[0 0 0]  RotationSequenceAnglesUnits=deg  RotationMatrix=[1 0 0; 0 1 0; 0 0 1]  Quaternion=[1 0 0 0]
  Rigid Transform (Setup Initial Disp) : sm_lib/Frames and Transforms/Rigid Transform  TranslationMethod=Cartesian  TranslationStandardOffset=0  TranslationLengthUnit=m  TranslationStandardAxis=+Z  TranslationCartesianOffset=body.initial.displacement  TranslationROffset=0  TranslationROffsetUnits=m  TranslationZOffset=0  TranslationZOffsetUnits=m  TranslationThetaOffset=0  TranslationThetaOffsetUnits=deg  RotationMethod=ArbitraryAxis  RotationAngleUnits=rad  RotationStandardAxis=+Y  RotationAngle=body.initial.angle  RotationArbitraryAxis=body.initial.axis  FollAlignAxisA=+X  BaseAlignAxisA=+Y  FollAlignAxisB=+Y  BaseAlignAxisB=+Z  RotationSequenceAxes=FollowerAxes  RotationSequence=XYX  RotationSequenceAngles=[0 0 0]  RotationSequenceAnglesUnits=deg  RotationMatrix=[1 0 0; 0 1 0; 0 0 1]  Quaternion=[1 0 0 0]
  Selector : Selector  InputPortWidth=6  IndexOptions=Index vector (dialog)  Indices=[1:3]  OutputSizes=1
  Selector1 : Selector  InputPortWidth=6  IndexOptions=Index vector (dialog)  Indices=[4:6]  OutputSizes=1
  Simulink-PS Converter1 : nesl_utility/Simulink-PS Converter  PhysicalDomain=network_engine_domain  SubClassName=ps_input  LeftPortType=input  RightPortType=output  PseudoPeriodic=off  Frequencies=[]  NoiseDistribution=none  NoiseParameters=[]  Unit=1  AffineConversion=off  FilteringAndDerivatives=zero  SimscapeFilterOrder=1  InputFilterTimeConstant=0.001  UdotUserProvided=1
  Simulink-PS Converter2 : nesl_utility/Simulink-PS Converter  PhysicalDomain=network_engine_domain  SubClassName=ps_input  LeftPortType=input  RightPortType=output  PseudoPeriodic=off  Frequencies=[]  NoiseDistribution=none  NoiseParameters=[]  Unit=1  AffineConversion=off  FilteringAndDerivatives=zero  SimscapeFilterOrder=1  InputFilterTimeConstant=0.001  UdotUserProvided=1
  World Frame : sm_lib/Frames and Transforms/World Frame
  Conn Free Surface : PMIOPort  Side=Right
  Response : Outport
  wires:
  Total Force/1 -> Selector1/1, Selector/1
  Selector/1 -> Simulink-PS Converter1/1
  Selector1/1 -> Simulink-PS Converter2/1
  Motion Sensor/1 -> Response/1
  connections:
  External Force and Torque/LConn1 -- Simulink-PS Converter1/RConn1
  External Force and Torque/LConn2 -- Simulink-PS Converter2/RConn1
  Rigid Transform (Setup Initial Disp)/RConn1 -- Body Properties/RConn1 -- External Force and Torque/RConn1 -- Motion Sensor/RConn1
  Conn Free Surface/RConn1 -- Rigid Transform (Setup CG)/LConn1
  Rigid Transform (Setup Initial Disp)/LConn1 -- Rigid Transform (Setup CG)/RConn1
  Motion Sensor/LConn1 -- World Frame/RConn1

== system WECSim_Lib_Body_Elements_2022b/Flex Body/Wave Diffraction and Excitation Force Calculation ==
  note: Do not link the `Wave Diffraction and Excitation Force Calculation`
      | to the rigid body block, this will break the Flex Body block.
  Time : Inport
  Displacement : Inport  Port=2
  WaveElv : Inport  Port=3
  Selector : Selector  InputPortWidth=body.dof  IndexOptions=Index vector (dialog)  Indices=[1:6]  OutputSizes=1
  Selector1 : Selector  InputPortWidth=body.dof  IndexOptions=Index vector (dialog)  Indices=[7:body.dofEnd]  OutputSizes=1
  Wave Diffraction and Excitation Force Calculation : Subsystem
  F_Excitation_Rigid : Outport  PortDimensions=6
  F_Excitation_Flex : Outport  Port=2  PortDimensions=body.gbmDOF
  wires:
  Wave Diffraction and Excitation Force Calculation/1(F_Excitation) -> Selector1/1, Selector/1
  Selector/1 -> F_Excitation_Rigid/1
  Selector1/1 -> F_Excitation_Flex/1
  Time/1 -> Wave Diffraction and Excitation Force Calculation/1(Time)
  WaveElv/1 -> Wave Diffraction and Excitation Force Calculation/3(WaveElv)
  Displacement/1 -> Wave Diffraction and Excitation Force Calculation/2(Displacement)

== system WECSim_Lib_Body_Elements_2022b/Flex Body/Wave Radiation Forces Calculation ==
  Velocity : Inport
  Acceleration : Inport  Port=2
  Selector : Selector  InputPortWidth=body.dof  IndexOptions=Index vector (dialog)  Indices=[1:6]  OutputSizes=1
  Selector1 : Selector  InputPortWidth=body.dof  IndexOptions=Index vector (dialog)  Indices=[7:body.dofEnd]  OutputSizes=1
  Selector2 : Selector  InputPortWidth=body.dof  IndexOptions=Index vector (dialog)  Indices=[1:6]  OutputSizes=1
  Selector3 : Selector  InputPortWidth=body.dof  IndexOptions=Index vector (dialog)  Indices=[7:body.dofEnd]  OutputSizes=1
  Wave Radiation Forces Calculation : $bdroot/Rigid Body/Hydrodynamic Body/Wave Radiation Forces Calculation  SystemSampleTime=-1  Latency=0  AutoFrameSizeCalculation=off
  F_RadiationDamping_Rigid : Outport  PortDimensions=6
  F_RadiationDamping_Flex : Outport  Port=2  PortDimensions=body.gbmDOF
  F_AddedMass_Rigid : Outport  Port=3  PortDimensions=6
  F_AddedMass_Flex : Outport  Port=4  PortDimensions=body.gbmDOF
  wires:
  Wave Radiation Forces Calculation/2 -> Selector3/1, Selector2/1  "F_AddedMass"
  Selector2/1 -> F_AddedMass_Rigid/1
  Selector3/1 -> F_AddedMass_Flex/1
  Selector/1 -> F_RadiationDamping_Rigid/1
  Selector1/1 -> F_RadiationDamping_Flex/1
  Wave Radiation Forces Calculation/1 -> Selector/1, Selector1/1  "F_RadiationDamping"
  Acceleration/1 -> Wave Radiation Forces Calculation/2
  Velocity/1 -> Wave Radiation Forces Calculation/1

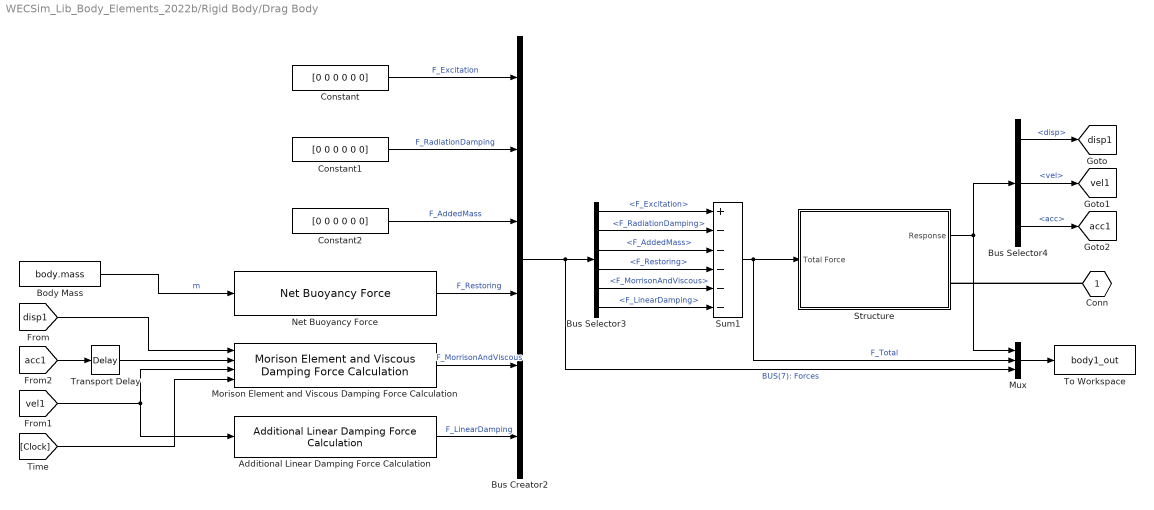
== system WECSim_Lib_Body_Elements_2022b/Rigid Body/Drag Body ==
  Additional Linear Damping Force Calculation : $bdroot/Rigid Body/Hydrodynamic Body/Additional Linear Damping Force Calculation  SystemSampleTime=-1  Latency=0  AutoFrameSizeCalculation=off
  Body Mass : Constant  Value=body.mass
  Bus Creator2 : BusCreator  Inputs=6
  Bus Selector3 : BusSelector  OutputSignals=F_Excitation,F_RadiationDamping,F_AddedMass,F_Restoring,F_MorrisonAndViscous,F_LinearDamping
  Bus Selector4 : BusSelector  OutputSignals=disp,vel,acc
  Constant : Constant  Value=[0 0 0 0 0 0]
  Constant1 : Constant  Value=[0 0 0 0 0 0]
  Constant2 : Constant  Value=[0 0 0 0 0 0]
  Morison Element and Viscous Damping Force Calculation : $bdroot/Rigid Body/Hydrodynamic Body/Morison Element and Viscous Damping Force Calculation  SystemSampleTime=-1  Latency=0  AutoFrameSizeCalculation=off
  Mux : Mux  Inputs=3
  Net Buoyancy Force : $bdroot/Rigid Body/Hydrodynamic Body/Hydrostatic Restoring Force Calculation/Linear and Nonlinear Restoring Force Variant Subsystem/Linear Hydrostatic Restoring Force/Net Buoyancy Force  SystemSampleTime=-1  Latency=0  AutoFrameSizeCalculation=off
  Structure : Subsystem
  Sum1 : Sum  Inputs=+-----
  To Workspace : ToWorkspace  VariableName=body1_out  SaveFormat=Structure With Time  SampleTime=simu.dtOut
  Transport Delay : TransportDelay  DelayTime=10e-8
  Conn : PMIOPort  Side=Right
  tag scope: acc1=global, disp1=global, vel1=global
  wires:
  [acc1] -> Transport Delay/1
  Bus Selector3/1 -> Sum1/1  "<F_Excitation>"
  Bus Selector3/5 -> Sum1/5  "<F_MorrisonAndViscous>"
  Constant1/1 -> Bus Creator2/2  "F_RadiationDamping"
  Mux/1 -> To Workspace/1
  Net Buoyancy Force/1 -> Bus Creator2/4  "F_Restoring"
  Additional Linear Damping Force Calculation/1 -> Bus Creator2/6  "F_LinearDamping"
  Morison Element and Viscous Damping Force Calculation/1 -> Bus Creator2/5  "F_MorrisonAndViscous"
  Constant/1 -> Bus Creator2/1  "F_Excitation"
  Bus Selector3/4 -> Sum1/4  "<F_Restoring>"
  Bus Selector3/3 -> Sum1/3  "<F_AddedMass>"
  Bus Creator2/1 -> Mux/3, Bus Selector3/1  "BUS(7): Forces"
  Sum1/1 -> Mux/2, Structure/1(Total Force)  "F_Total"
  Constant2/1 -> Bus Creator2/3  "F_AddedMass"
  Bus Selector3/2 -> Sum1/2  "<F_RadiationDamping>"
  Bus Selector3/6 -> Sum1/6  "<F_LinearDamping>"
  Bus Selector4/1 -> [disp1]  "<disp>"
  Bus Selector4/2 -> [vel1]  "<vel>"
  Structure/1(Response) -> Mux/1, Bus Selector4/1
  Bus Selector4/3 -> [acc1]  "<acc>"
  Transport Delay/1 -> Morison Element and Viscous Damping Force Calculation/2
  [vel1] -> Morison Element and Viscous Damping Force Calculation/3, Additional Linear Damping Force Calculation/1
  [Clock] -> Morison Element and Viscous Damping Force Calculation/4
  [disp1] -> Morison Element and Viscous Damping Force Calculation/1
  Body Mass/1 -> Net Buoyancy Force/1  "m"
  connections:
  Conn/RConn1 -- Structure/RConn1
